simulink model "clik_inverse"  (R2022b)
settings: Solver=ode1  StartTime=0.0  StopTime=4  FixedStep=0.001  RelTol=1e-3
undefined symbols (not defined in the file or in its folder): DiscIntNeverNeededParam, q0, Tc
settings Model: Creator=Xp  LastModifiedBy=DELL
settings SolverCC: AlgebraicLoopSolver=TrustRegion
settings DataIOCC: LimitDataPoints=on  SaveFormat=Array  SignalLoggingSaveFormat=ModelDataLogs  ReturnWorkspaceOutputs=off
settings OptimizationCC: ExpressionDepthLimit=2147483647  InitFltsAndDblsToZero=on  LifeSpan=inf
settings DebuggingCC: SaveWithParameterizedLinksMsg=none  UnderspecifiedInitializationDetection=Classic  MergeDetectMultiDrivingBlocksExec=none  SolverPrmCheckMsg=warning  MultiTaskDSMMsg=warning  MultiTaskCondExecSysMsg=none  FcnCallInpInsideContextMsg=warning  UnconnectedInputMsg=warning  UnconnectedOutputMsg=warning  UnconnectedLineMsg=warning  StateNameClashWarn=warning  SFUnexpectedBacktrackingDiag=warning  SFNoUnconditionalDefaultTransitionDiag=warning  SFExecutionAtInitializationDiag=none  SFMachineParentedDataDiag=warning  ArithmeticOperatorsInVariantConditions=warning
settings HardwareCC: ProdBitPerPointer=32  ProdBitPerSizeT=32  ProdBitPerPtrDiffT=32  ProdLargestAtomicFloat=None  ProdIntDivRoundTo=Undefined  ProdEndianess=Unspecified  ProdWordSize=32  ProdHWDeviceType=32-bit Generic
settings ModelReferenceCC: EnableRefExpFcnMdlSchedulingChecks=on  PropagateSignalLabelsOutOfModel=off
settings SFSimCC: CustomCodeUndefinedFunction=UseInterfaceOnly
settings RTWCC: DLArmComputeVersion=19.05
settings CodeAppCC: StateflowObjectComments=on
settings GRTTargetCC: TargetLangStandard=C89/C90 (ANSI)  CombineOutputUpdateFcns=off  GRTInterface=on
settings ConfigComp: CovMetricSettings=dw  CovSaveCumulativeToWorkspaceVar=on  CovSaveSingleToWorkspaceVar=on

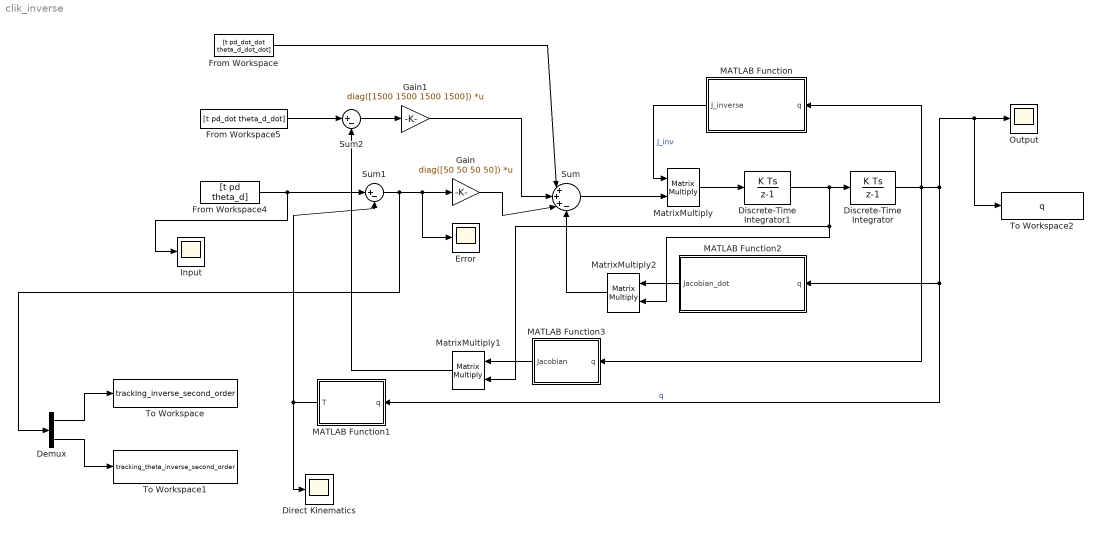
== system clik_inverse ==
  Demux : Demux  Outputs=2
  Direct Kinematics : Scope
  Discrete-Time Integrator : DiscreteIntegrator  InitialCondition=q0  SampleTime=Tc  LimitOutput=on  UpperSaturationLimit=[pi/2;pi/4;1;2*pi]  LowerSaturationLimit=[-pi/2;-pi/2;0.25;-2*pi]  ICPrevOutput=DiscIntNeverNeededParam  ICPrevScaledInput=DiscIntNeverNeededParam
  Discrete-Time Integrator1 : DiscreteIntegrator  SampleTime=Tc  UpperSaturationLimit=[pi/2;pi/4;1;2*pi]  LowerSaturationLimit=[-pi/2;-pi/2;0.25;-2*pi]  ICPrevOutput=DiscIntNeverNeededParam  ICPrevScaledInput=DiscIntNeverNeededParam
  Error : Scope
  From Workspace : FromWorkspace  VariableName=[t pd_dot_dot theta_d_dot_dot]  SampleTime=Tc
  From Workspace4 : FromWorkspace  VariableName=[t pd theta_d]  SampleTime=Tc
  From Workspace5 : FromWorkspace  VariableName=[t pd_dot theta_d_dot]  SampleTime=Tc
  Gain : Gain  Gain=diag([50 50 50 50])  Multiplication=Matrix(K*u)
  Gain1 : Gain  Gain=diag([1500 1500 1500 1500])  Multiplication=Matrix(K*u)
  Input : Scope
  MATLAB Function : MATLAB Function  TreatAsAtomicUnit=on
  MATLAB Function1 : MATLAB Function  TreatAsAtomicUnit=on
  MATLAB Function2 : MATLAB Function  TreatAsAtomicUnit=on
  MATLAB Function3 : MATLAB Function  TreatAsAtomicUnit=on
  MatrixMultiply : Product  Multiplication=Matrix(*)
  MatrixMultiply1 : Product  Multiplication=Matrix(*)
  MatrixMultiply2 : Product  Multiplication=Matrix(*)
  Output : Scope
  Sum : Sum  Inputs=|+++-
  Sum1 : Sum  Inputs=|+-
  Sum2 : Sum  Inputs=|+-
  To Workspace : ToWorkspace  VariableName=tracking_inverse_second_order  SampleTime=Tc
  To Workspace1 : ToWorkspace  VariableName=tracking_theta_inverse_second_order  SampleTime=Tc
  To Workspace2 : ToWorkspace  VariableName=q  SampleTime=Tc
  wires:
  MatrixMultiply/1 -> Discrete-Time Integrator1/1
  Sum/1 -> MatrixMultiply/2
  Sum1/1 -> Demux/1, Error/1, Gain/1
  From Workspace4/1 -> Input/1, Sum1/1
  MATLAB Function1/1(T) -> Direct Kinematics/1, Sum1/2
  Discrete-Time Integrator/1 -> MATLAB Function3/1(q), MATLAB Function/1(q), MATLAB Function2/1(q), MATLAB Function1/1(q), To Workspace2/1, Output/1  "q"
  MATLAB Function/1(J_inverse) -> MatrixMultiply/1  "J_inv"
  Gain/1 -> Sum/3
  From Workspace/1 -> Sum/1
  From Workspace5/1 -> Sum2/1
  Sum2/1 -> Gain1/1
  Gain1/1 -> Sum/2
  Discrete-Time Integrator1/1 -> MatrixMultiply2/2, MatrixMultiply1/2, Discrete-Time Integrator/1
  MatrixMultiply2/1 -> Sum/4
  MatrixMultiply1/1 -> Sum2/2
  MATLAB Function3/1(Jacobian) -> MatrixMultiply1/1
  MATLAB Function2/1(Jacobian_dot) -> MatrixMultiply2/1
  Demux/1 -> To Workspace/1
  Demux/2 -> To Workspace1/1

== matlab function clik_inverse/MATLAB Function1 ==
  data: q input; T output
function T = direct_kin(q)

% Defining link length values
a1 = 0.5;
a2 = 0.5;
d0 = 1;

% Assigning individual joint values to the corresponding rows of the
% q(angle) being taken as input
q1=q(1);
q2=q(2);
d3=q(3);
q4=q(4);

% Obtained Rotation and translation direct kinematics matrix for scara manipulator
R=[cos(q1+q2+q4),sin(q1+q2+q4),0;sin(q1+q2+q4),-cos(q1+q2+q4),0;0,0,-1;0 0 0];
T=[a1*cos(q1)+a2*cos(q1+q2);a1*sin(q1)+a2*sin(q1+q2);-d3+d0;q1+q2+q4];

== matlab function clik_inverse/MATLAB Function ==
  data: q input; J_inverse output
function J_inverse = jacobian_inverse(q)

% Calling the jacobian function from the jacobian matlab file
J = jacobian(q);

% Calculating inverse of jacobian matrix
J_inverse = inv(J);

== matlab function clik_inverse/MATLAB Function2 ==
  data: q input; Jacobian_dot output
function Jacobian_dot = jacobian_dot(q)

% Calling the jacobian_dot function which finds first order differential of
% jacobian matrix
Jacobian_dot = jacobian_dot(q);

== matlab function clik_inverse/MATLAB Function3 ==
  data: q input; Jacobian output
function Jacobian = jacobian(q)

% Caling the jacobian function to get the jacobian matrix
Jacobian = jacobian(q);
